simulink model "simulacion_logical"  (R2021b)
settings: Solver=VariableStepAuto  StartTime=0.0  StopTime=10.0  RelTol=1e-3
settings Model: Creator=Alumno103  LastModifiedBy=Alumno103

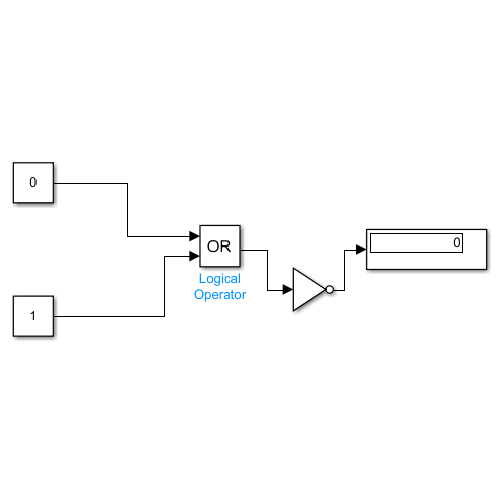
[thumbnail: Simulink's stored preview of the top-level diagram]
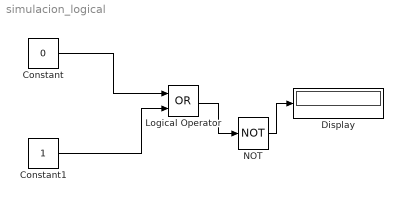
== system simulacion_logical ==
  Constant : Constant  Value=0
  Constant1 : Constant
  Display : Display
  Logical Operator : Logic  Operator=OR  AllPortsSameDT=off  OutDataTypeStr=boolean
  NOT : Logic  Operator=NOT  IconShape=distinctive  AllPortsSameDT=off  OutDataTypeStr=boolean
  wires:
  Constant/1 -> Logical Operator/1
  Constant1/1 -> Logical Operator/2
  Logical Operator/1 -> NOT/1
  NOT/1 -> Display/1
